simulink model "Modelisation_1_MGD_comparaison_avec_Clavel"  (R2016a)
settings: Solver=ode45  StartTime=0.0  StopTime=0  RelTol=1e-3
undefined symbols (not defined in the file or in its folder): sfun3d
settings Model: Creator=user  LastModifiedBy=NAD
settings DataIOCC: LimitDataPoints=on  SaveFormat=Array
settings HardwareCC: ProdBitPerPointer=32  ProdLargestAtomicFloat=None  ProdIntDivRoundTo=Undefined  ProdEndianess=Unspecified  ProdWordSize=32  ProdHWDeviceType=32-bit Generic
settings ModelReferenceCC: PropagateSignalLabelsOutOfModel=off
settings ConfigComp: CovModelRefEnable=Off

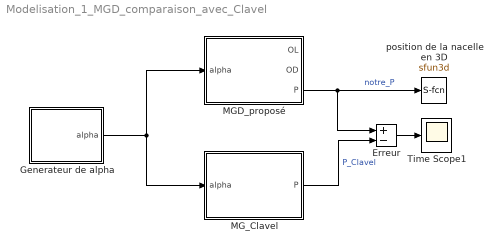
== system Modelisation_1_MGD_comparaison_avec_Clavel ==
  Erreur : Sum  Inputs=+-
  Generateur de alpha : Subsystem
  MGD_proposé : MATLAB Function  TreatAsAtomicUnit=on
  MG_Clavel : MATLAB Function  TreatAsAtomicUnit=on
  Time Scope1 : Scope
  "position de la nacelle en 3D " : S-Function  LoadFcn=sfun3d([],[],[],'LoadBlock')  StartFcn=sfun3d([],[],[],'Start')  StopFcn=sfun3d([],[],[],'Stop')  FunctionName=sfun3d  Parameters=ax,T,np,cp,gd,ls,mk  SFunctionDeploymentMode=off  EnableBusSupport=off  mask(3D Graph){np=1, ax=[-1 1 -1 1 -2 0]*0.3, cp=[3 2 1], gd=on, ls=-, mk=o, T=0.001}
      mask prompts: np "Number of point (lines)"; ax "[xmin xmax  ymin ymax zmin zmax]"; cp "Camera position (use [0 0 1] for 2D XY view)"; gd "Grid (on|off)"; ls "LineStyle"; mk "Marker"; T "Sampling Time"
      mask help:
      | This block plots the position of several points in the XYZ space. The input contains the coordinates of all the points (x1,y1,z1,x2,y2,z2,...).
      | The number of points (lines), the XYZ ranges, camera position, grid, linestyle, marker and sampling time, can be set as mask parameters.
      settings: CopyFcn=sfun3d([],[],[],'CopyBlock')  DeleteFcn=sfun3d([],[],[],'DeleteBlock')  NameChangeFcn=sfun3d([],[],[],'NameChange')
      mask Help:
      | This block plots the position of several points in the XYZ space. The input contains the coordinates of all the points (x1,y1,z1,x2,y2,z2,...).
      | The number of points (lines), the XYZ ranges, camera position, grid, linestyle, marker and sampling time, can be set as mask parameters.
      mask TypeOptions ls: - | -- | : | -. | none
      mask TypeOptions mk: none | . | + | o | * | x | square | diamond | v | ^ | > | < | pentagram | hexagram
      mask Display: plot([.05 .95 .95 .05 .05],[.45 .45 .95 .95 .45], 0.5+cos(0:0.1:2*pi)*0.3,0.7+sin(0:0.1:2*pi)*0.2)
  wires:
  MG_Clavel/1(P) -> Erreur/2  "P_Clavel"
  Generateur de alpha/1(alpha) -> MGD_proposé/1(alpha), MG_Clavel/1(alpha)
  MGD_proposé/3(P) -> Erreur/1, "position de la nacelle en 3D "/1  "notre_P"
  Erreur/1 -> Time Scope1/1

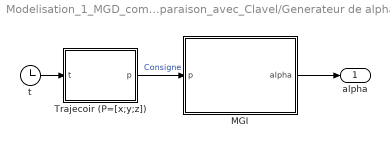
== system Modelisation_1_MGD_comparaison_avec_Clavel/Generateur de alpha ==
  MGI : MATLAB Function  TreatAsAtomicUnit=on
  Trajecoir (P=[x;y;z]) : MATLAB Function  TreatAsAtomicUnit=on
  t : Clock
  alpha : Outport
  wires:
  t/1 -> Trajecoir (P=[x;y;z])/1(t)
  Trajecoir (P=[x;y;z])/1(p) -> MGI/1(p)  "Consigne"
  MGI/1(alpha) -> alpha/1

== matlab function Modelisation_1_MGD_comparaison_avec_Clavel/MG_Clavel ==
  data: alpha input; P output
function P = MGD(alpha)


alpha1=alpha(1) ;alpha2=alpha(2) ; alpha3=alpha(3) ;
%% les constantes :
l1 = 0.19992; 
l2 = 0.334; 
r = 0.126; 
phi1 = 0 ;
phi2 = 2*pi/3;
phi3 = 4*pi/3;

 D1 = -l2^2 + l1^2 + r^2 + 2*r*l1*cos(alpha1);
 D2 = -l2^2 + l1^2 + r^2 + 2*r*l1*cos(alpha2);
 D3 = -l2^2 + l1^2 + r^2 + 2*r*l1*cos(alpha3);

 E1 = 2*(r + l1*cos(alpha1))*cos(phi1);
 E2 = 2*(r + l1*cos(alpha2))*cos(phi2);
 E3 = 2*(r + l1*cos(alpha3))*cos(phi3);

 F1 = 2*(r + l1*cos(alpha1))*sin(phi1);
 F2 = 2*(r + l1*cos(alpha2))*sin(phi2);
 F3 = 2*(r + l1*cos(alpha3))*sin(phi3);

 G1 = -2*l1*sin(alpha1);
 G2 = -2*l1*sin(alpha2);
 G3 = -2*l1*sin(alpha3);

 H1 = -(E3 - E1)*(G2 - G1) + (G3 - G1)*(E2 - E1);
 H2 = -(F3 - F1)*(E2 - E1) + (E3 - E1)*(F2 - F1);
 H3 = -(D3 - D1)*(E2 - E1) + (E3 - E1)*(D2 - D1);
 H4 = (D3 - D1)*(F2 - F1) + (F3 - F1)*(D1 - D2);
 H5 = -(G3 - G1)*(F2 - F1) - (F3 - F1)*(G1 - G2);

 L = 1 + (H5^2 + H1^2)/H2^2;
 M = -2*(H5*H4 + H1*H3)/H2^2 + (E1*H5 + F1*H1)/H2 + G1;
 N = D1 + (H4^2 + H3^2)/H2^2 - (E1*H4 + F1*H3)/H2;

z = (M - sqrt(M^2 - 4*L*N))/(2*L);
x = (H5/H2)*z + H4/H2;
y = (H1/H2)*z + H3/H2;

P=[x;y;z];

== matlab function Modelisation_1_MGD_comparaison_avec_Clavel/Generateur de alpha/MGI ==
  data: p input; alpha output
function alpha = MGI(p)

l1 = 0.19992; 
l2 = 0.334; 
r = 0.126; 
phi2 = 2*pi/3;
phi3 = 4*pi/3;

%% projection de P sur Ri
A2=[cos(phi2) sin(phi2) 0
    -sin(phi2) cos(phi2) 0
    0            0      1 ]; 
A3=[cos(phi3) sin(phi3) 0
    -sin(phi3) cos(phi3) 0
    0            0      1 ];
p2=A2*p; p3=A3*p ;

x1=p(1); y1=p(2) ; z1=p(3) ; %% p1=p
x2=p2(1); y2=p2(2) ; z2=p2(3) ;
x3=p3(1); y3=p3(2) ; z3=p3(3) ;

%% Calcule de ABi et ei :
AB1=sqrt(z1^2+(x1-r)^2);
e1=sqrt(l2^2-y1^2); 
AB2=sqrt(z2^2+(x2-r)^2);
e2=sqrt(l2^2-y2^2);
AB3=sqrt(z3^2+(x3-r)^2);
e3=sqrt(l2^2-y3^2);

%% calcul de alpha1
beta1=atan2(-z1,x1-r);
gama1=acos((AB1^2 + l1^2 - e1^2)/(2*l1*AB1));
alpha11=beta1-gama1; 
alpha12=beta1+gama1; 

%% calcul de alpha2
beta2=atan2(-z2,x2-r);
gama2=acos((AB2^2 + l1^2 - e2^2)/(2*l1*AB2));
alpha21=beta2-gama2; 
alpha22=beta2+gama2; 

%% calcul de alpha3
beta3=atan2(-z3,x3-r);
gama3=acos((AB3^2 + l1^2 - e3^2)/(2*l1*AB3));
alpha31=beta3-gama3; 
alpha32=beta3+gama3; 

%% Premiere Solution, Deuxieme Solution :
alpha=[alpha11;alpha21;alpha31];
% solution2=[alpha12,alpha22,alpha32];

== matlab function Modelisation_1_MGD_comparaison_avec_Clavel/MGD_proposé ==
  data: OL output; OD output; alpha input; P output
function [OL,OD,P] =MGD(alpha)

alpha1=alpha(1) ;alpha2=alpha(2) ; alpha3=alpha(3) ;

%les constantes
l1 = 0.19992; 
l2 = 0.334; 
r = 0.126; 
phi2 = 2*pi/3;
phi3 = 4*pi/3;

%% Les points :
C1=[r+l1*cos(alpha1) ; 0 ; -l1*sin(alpha1) ]; 
C2=[(r+l1*cos(alpha2))*cos(phi2) ; (r+l1*cos(alpha2))*sin(phi2) ; -l1*sin(alpha2) ]; 
C3=[(r+l1*cos(alpha3))*cos(phi3) ; (r+l1*cos(alpha3))*sin(phi3) ; -l1*sin(alpha3) ]; 

%% Les vecteurs du triangle C1C2C3 et ses distances
C1C2= C2-C1 ; C2C3 =C3-C2 ; C3C1= C1-C3 ;
a=sqrt(C1C2'*C1C2) ; b=sqrt(C2C3'*C2C3)  ; c=sqrt(C3C1'*C3C1)  ;
 p= a+b+c ; % Le perimetre de C1C2C3
 R = a*b*c/sqrt(p*(p-2*a)*(p-2*b)*(p-2*c)) ;

 %% Calcule du point L 
 % Les vecteurs u et n:
 v1=C1C2/a ;
 n=cross(C3C1,C1C2)*2*R/(a*b*c) ;
 OT = (C1+C2)/2 ;
 tl = sqrt(R^2-a^2/4) ;
 TL=sign(-a*a+c*c+b*b)*tl*cross(n,v1);
  OL=OT+TL;
 %% Calcule du point E :
P=OL-sqrt(l2^2-R^2)*n ; 

%% Calculating of OD:
H=[ C1C2'*[C1 C2 C3]
    C1C3'*[C1 C2 C3]
    1      1     1   ];
N=[(a^2-b^2)/2 ; (a^2-c^2)/2 ; 1 ];
OD = H\N ;

== matlab function Modelisation_1_MGD_comparaison_avec_Clavel/Generateur de alpha/Trajecoir (P=[x;y;z]) ==
  data: t input; p output
function p = fcn(t)
 
f = 3; 
R=0.25;
x=R*cos(f*t) ; y=R*sin(f*t) ; z=-0.35;

p=[x ; y ; z];
